simulink model "Simu_ControlLoop_FixPt"  (Simulink 9.2)
settings: Solver=VariableStepAuto  StartTime=0.0  StopTime=25  MaxStep=50e-6  RelTol=1e-3
PreLoadFcn:
  | InitTPV0;
values from neighbouring files (symbols this model uses):
  Imax = 4.4    [InitTPV0.m]
  Kelec = -place(Ae,Be,Pole_elec_desiree)    [InitTPV0.m]
  Kmeca = place(Am,Bm,Pole_meca_desiree)    [InitTPV0.m]
  Ts = 50e-6    (= 5e-05)    [InitTPV0.m]
  Vmax = 24    [InitTPV0.m]
  Wmax = 350    [InitTPV0.m]
undefined symbols (not defined in the file or in its folder): DiscIntNeverNeededParam
libraries: simulink x1
settings Model: Creator=romaindelpoux  LastModifiedBy=rdelpoux
settings SolverCC: ZeroCrossControl=DisableAll  AlgebraicLoopSolver=LineSearch
settings DataIOCC: LimitDataPoints=off  SaveFormat=Dataset  SignalLoggingSaveFormat=Dataset
settings OptimizationCC: LifeSpan=auto
settings DebuggingCC: UnderspecifiedInitializationDetection=Simplified  MergeDetectMultiDrivingBlocksExec=error  FcnCallInpInsideContextMsg=error  StateNameClashWarn=none  SFUnexpectedBacktrackingDiag=error  SFNoUnconditionalDefaultTransitionDiag=error  SFExecutionAtInitializationDiag=warning
settings HardwareCC: ProdBitPerPointer=64  ProdBitPerSizeT=64  ProdBitPerPtrDiffT=64  ProdLargestAtomicFloat=Float  ProdIntDivRoundTo=Zero  ProdEndianess=LittleEndian  ProdWordSize=64  ProdHWDeviceType=Intel->x86-64 (Windows64)
settings ModelReferenceCC: PropagateSignalLabelsOutOfModel=on
settings CodeAppCC: StateflowObjectComments=off
settings GRTTargetCC: TargetLangStandard=C99 (ISO)  GeneratePreprocessorConditionals=Use local settings  CombineOutputUpdateFcns=on  GRTInterface=off
settings ConfigComp: CovMetricSettings=dwe  CovHtmlReporting=off  CovSaveCumulativeToWorkspaceVar=off  CovSaveSingleToWorkspaceVar=off  CovExternalEMLEnable=on

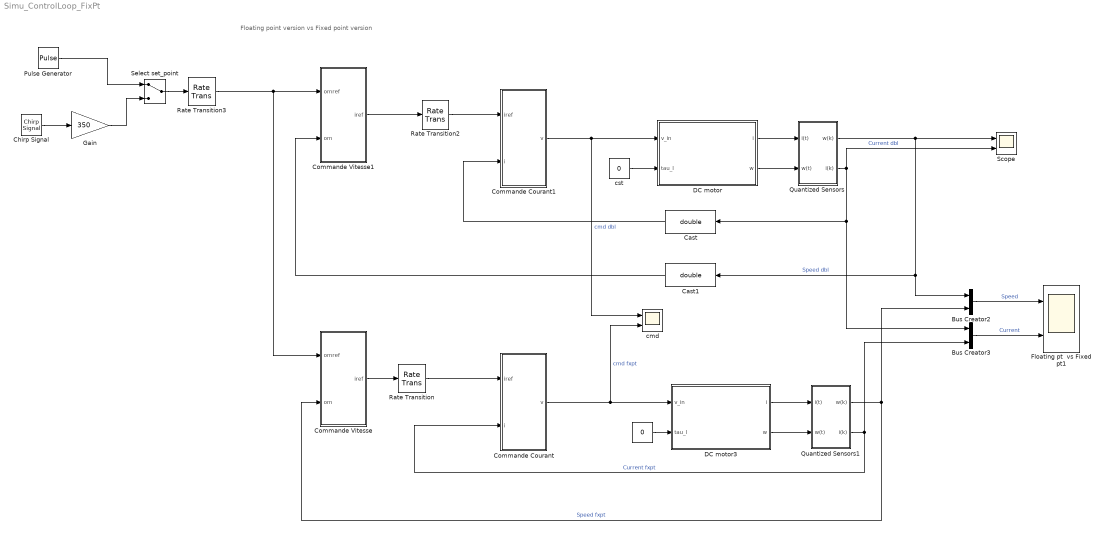
== system Simu_ControlLoop_FixPt ==
  note: Floating point version vs Fixed point version
  " " : Constant  Value=0  OutDataTypeStr=Inherit: Inherit via back propagation
  Bus Creator2 : BusCreator  Inputs=2
  Bus Creator3 : BusCreator  Inputs=2
  Cast : DataTypeConversion  OutDataTypeStr=double
  Cast1 : DataTypeConversion  OutDataTypeStr=double
  Chirp Signal : simulink/Sources/Chirp Signal  f1=0.1  T=20  f2=5
  Commande Courant : Subsystem
  Commande Courant1 : Subsystem
  Commande Vitesse : Subsystem
  Commande Vitesse1 : Subsystem
  DC motor : Subsystem  mask(Motor PRAVALUX MPM4-0002){R=1.22, L=0.0027, Kphi=0.061, J=0.22e-3, F=.0001, C0=-0.032, mod=0.25*0}
      mask prompts: R "Resistance (R) in Ohms"; L "Inductance (L) in H"; Kphi "Back EMF (Kphi) in V/rad/s"; J "J in kgm²"; F "F in N/rad/s"; mod "BEMF modulation (default: 0.25, 0 for off)"
      mask help:
      | Continuous time Model for PRAVALUX MPM4 DC motor
      | Caracteristics: 24V DC, 90W, 5.2A, 3000RPM
      |
      | It is a 2nd order model made of two intertwinned system:
      | one 1st order electrical system and one 1st order mechanical system.
      |
      | Modulation on the BEMF can be added to fit with motor current ripple measured
      |
      | Look under mask (Ctrl-U) to see the model
      mask Display:
      | color('green');
      | image('MotorPravalux.png');
      | %port_label('input',1,'DC');
      | %port_label('output',1,'BEMF');
  DC motor3 : Subsystem  mask(Motor PRAVALUX MPM4-0002){R=1.22, L=0.0027, Kphi=0.061, J=0.22e-3, F=.0001, C0=-0.032, mod=0.25*0}
      mask prompts: R "Resistance (R) in Ohms"; L "Inductance (L) in H"; Kphi "Back EMF (Kphi) in V/rad/s"; J "J in kgm²"; F "F in N/rad/s"; mod "BEMF modulation (default: 0.25, 0 for off)"
      mask help:
      | Continuous time Model for PRAVALUX MPM4 DC motor
      | Caracteristics: 24V DC, 90W, 5.2A, 3000RPM
      |
      | It is a 2nd order model made of two intertwinned system:
      | one 1st order electrical system and one 1st order mechanical system.
      |
      | Modulation on the BEMF can be added to fit with motor current ripple measured
      |
      | Look under mask (Ctrl-U) to see the model
      mask Display:
      | color('green');
      | image('MotorPravalux.png');
      | %port_label('input',1,'DC');
      | %port_label('output',1,'BEMF');
  Floating pt  vs Fixed pt1 : Scope  NumInputPorts=2
  Gain : Gain  Gain=350  OutDataTypeStr=Inherit: Inherit via back propagation
  Pulse Generator : DiscretePulseGenerator  PulseType=Time based  Amplitude=200  PulseWidth=50  PhaseDelay=0.5  SampleTime=-1
  Quantized Sensors : Subsystem
  Quantized Sensors1 : Subsystem
  Rate Transition : RateTransition  Deterministic=off  OutPortSampleTime=50e-6
  Rate Transition2 : RateTransition  Deterministic=off
  Rate Transition3 : RateTransition  Deterministic=off
  Scope : Scope  NumInputPorts=2
  Select set_point : ManualSwitch
  cmd : Scope  NumInputPorts=2
  cst : Constant  Value=0
  wires:
  Commande Vitesse/1(iref) -> Rate Transition/1
  DC motor3/1(i) -> Quantized Sensors1/1(i(t))
  DC motor3/2(w) -> Quantized Sensors1/2(w(t))
  Rate Transition/1 -> Commande Courant/1(iref)
  " "/1 -> DC motor3/2(tau_l)
  Rate Transition2/1 -> Commande Courant1/1(iref)
  Cast/1 -> Commande Courant1/2(i)
  Cast1/1 -> Commande Vitesse1/2(om)
  Rate Transition3/1 -> Commande Vitesse/1(omref), Commande Vitesse1/1(omref)
  DC motor/1(i) -> Quantized Sensors/1(i(t))
  Commande Vitesse1/1(iref) -> Rate Transition2/1
  Pulse Generator/1 -> Select set_point/1
  Select set_point/1 -> Rate Transition3/1
  Gain/1 -> Select set_point/2
  cst/1 -> DC motor/2(tau_l)
  DC motor/2(w) -> Quantized Sensors/2(w(t))
  Chirp Signal/1 -> Gain/1
  Bus Creator3/1 -> Floating pt  vs Fixed pt1/2  "Current"
  Bus Creator2/1 -> Floating pt  vs Fixed pt1/1  "Speed"
  Quantized Sensors/2(i(k)) -> Bus Creator3/1, Cast/1, Scope/2  "Current dbl"
  Quantized Sensors/1(w(k)) -> Bus Creator2/1, Cast1/1, Scope/1  "Speed dbl"
  Quantized Sensors1/2(i(k)) -> Bus Creator3/2, Commande Courant/2(i)  "Current fxpt"
  Quantized Sensors1/1(w(k)) -> Bus Creator2/2, Commande Vitesse/2(om)  "Speed fxpt"
  Commande Courant1/1(v) -> cmd/1, DC motor/1(v_in)  "cmd dbl"
  Commande Courant/1(v) -> cmd/2, DC motor3/1(v_in)  "cmd fxpt"

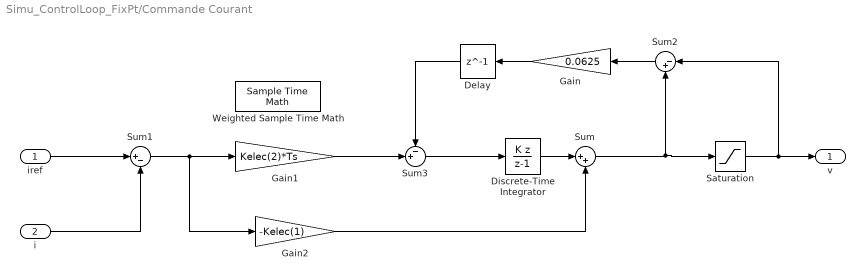
== system Simu_ControlLoop_FixPt/Commande Courant ==
  iref : Inport
  i : Inport  Port=2
  Delay : Delay  DelayLength=1  InitialCondition=0
  Discrete-Time Integrator : DiscreteIntegrator  IntegratorMethod=Accumulation: Backward Euler  SampleTime=.00005  OutMax=Vmax*2  OutDataTypeStr=fixdt(1,32)  SaturateOnIntegerOverflow=on  ICPrevOutput=DiscIntNeverNeededParam  ICPrevScaledInput=DiscIntNeverNeededParam
  Gain : Gain  Gain=0.0625  OutDataTypeStr=Inherit: Inherit via back propagation  SaturateOnIntegerOverflow=on
  Gain1 : Gain  Gain=Kelec(2)*Ts  OutMax=2*Imax*Kelec(2)*Ts  OutDataTypeStr=fixdt(1,16)  SaturateOnIntegerOverflow=on
  Gain2 : Gain  Gain=-Kelec(1)  OutMax=Vmax  OutDataTypeStr=fixdt(1,16)  SaturateOnIntegerOverflow=on
  Saturation : Saturate  UpperLimit=Vmax  LowerLimit=-Vmax
  Sum : Sum  Inputs=|++  OutMax=Vmax*2  OutDataTypeStr=fixdt(1,16)  SaturateOnIntegerOverflow=on
  Sum1 : Sum  Inputs=|+-  OutDataTypeStr=fixdt(1,16,12)  SaturateOnIntegerOverflow=on
  Sum2 : Sum  Inputs=|-+  OutDataTypeStr=Inherit: Same as first input
  Sum3 : Sum  Inputs=-+|  OutDataTypeStr=Inherit: Same as accumulator  SaturateOnIntegerOverflow=on  InputSameDT=on
  Weighted Sample Time Math : SampleTimeMath  TsampMathOp=*  weightValue=Kelec(2)  TsampMathImp=Offline Scaling Adjustment
  v : Outport
  wires:
  iref/1 -> Sum1/1
  i/1 -> Sum1/2
  Sum1/1 -> Gain1/1, Gain2/1
  Gain1/1 -> Sum3/2
  Gain2/1 -> Sum/2
  Sum/1 -> Saturation/1, Sum2/2
  Saturation/1 -> v/1, Sum2/1
  Discrete-Time Integrator/1 -> Sum/1
  Sum3/1 -> Discrete-Time Integrator/1
  Sum2/1 -> Gain/1
  Gain/1 -> Delay/1
  Delay/1 -> Sum3/1

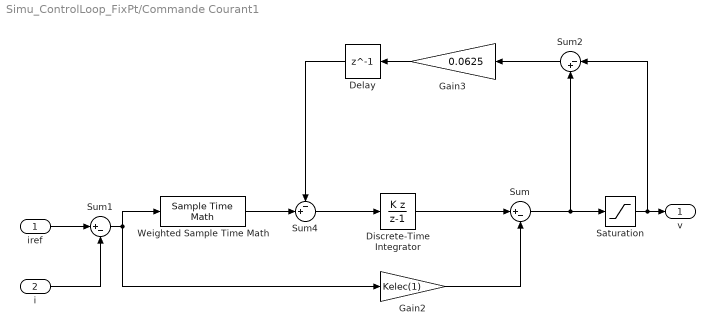
== system Simu_ControlLoop_FixPt/Commande Courant1 ==
  iref : Inport
  i : Inport  Port=2
  Delay : Delay  DelayLength=1  InitialCondition=0
  Discrete-Time Integrator : DiscreteIntegrator  IntegratorMethod=Accumulation: Backward Euler  SampleTime=-1  ICPrevOutput=DiscIntNeverNeededParam  ICPrevScaledInput=DiscIntNeverNeededParam
  Gain2 : Gain  Gain=Kelec(1)
  Gain3 : Gain  Gain=0.0625
  Saturation : Saturate  UpperLimit=Vmax  LowerLimit=-Vmax
  Sum : Sum  Inputs=|+-
  Sum1 : Sum  Inputs=|+-
  Sum2 : Sum  Inputs=|-+  OutDataTypeStr=Inherit: Same as accumulator
  Sum4 : Sum  Inputs=-+|
  Weighted Sample Time Math : SampleTimeMath  TsampMathOp=*  weightValue=Kelec(2)  TsampMathImp=Offline Scaling Adjustment
  v : Outport
  wires:
  Saturation/1 -> v/1, Sum2/1
  Sum/1 -> Saturation/1, Sum2/2
  iref/1 -> Sum1/1
  i/1 -> Sum1/2
  Gain2/1 -> Sum/2
  Sum1/1 -> Gain2/1, Weighted Sample Time Math/1
  Sum4/1 -> Discrete-Time Integrator/1
  Gain3/1 -> Delay/1
  Delay/1 -> Sum4/1
  Discrete-Time Integrator/1 -> Sum/1
  Sum2/1 -> Gain3/1
  Weighted Sample Time Math/1 -> Sum4/2

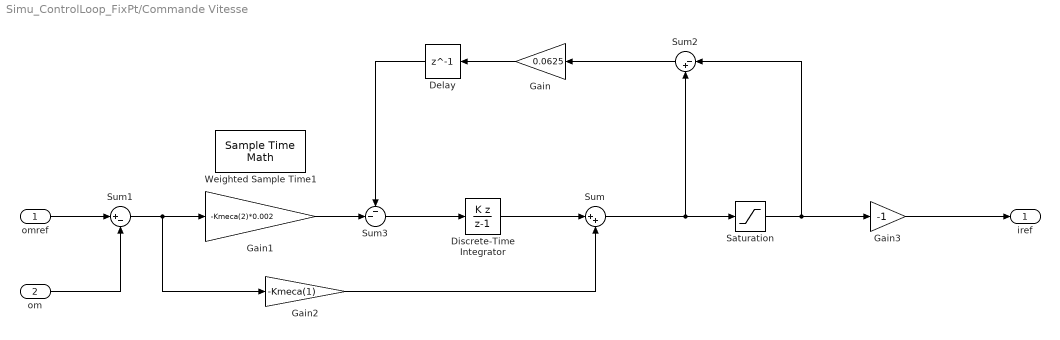
== system Simu_ControlLoop_FixPt/Commande Vitesse ==
  omref : Inport  OutMax=Wmax  OutDataTypeStr=fixdt(1,16)
  om : Inport  Port=2
  Delay : Delay  DelayLength=1  InitialCondition=0
  Discrete-Time Integrator : DiscreteIntegrator  IntegratorMethod=Accumulation: Backward Euler  SampleTime=.002  OutMin=0  OutMax=Imax*2  OutDataTypeStr=fixdt(1,32)  SaturateOnIntegerOverflow=on  ICPrevOutput=DiscIntNeverNeededParam  ICPrevScaledInput=DiscIntNeverNeededParam
  Gain : Gain  Gain=0.0625  OutDataTypeStr=Inherit: Inherit via back propagation  SaturateOnIntegerOverflow=on
  Gain1 : Gain  Gain=-Kmeca(2)*0.002  OutMin=0  OutMax=abs(Wmax * Kmeca(2) * 0.002)  OutDataTypeStr=fixdt(1,16)
  Gain2 : Gain  Gain=-Kmeca(1)  OutMin=-Imax*2  OutMax=Imax*2  OutDataTypeStr=fixdt(1,16)  SaturateOnIntegerOverflow=on
  Gain3 : Gain  Gain=-1  OutMin=-Imax  OutMax=Imax  SaturateOnIntegerOverflow=on  OutDataTypeStr=Inherit: Same as input
  Saturation : Saturate  UpperLimit=Imax  LowerLimit=-Imax
  Sum : Sum  Inputs=|++  OutMin=-Imax  OutMax=Imax*2  OutDataTypeStr=fixdt(1,16)  SaturateOnIntegerOverflow=on
  Sum1 : Sum  Inputs=|+-  OutMin=-Wmax*2  OutMax=Wmax*2  OutDataTypeStr=fixdt(1,16)
  Sum2 : Sum  Inputs=|-+  OutDataTypeStr=Inherit: Same as accumulator
  Sum3 : Sum  Inputs=--|  OutDataTypeStr=Inherit: Same as accumulator  SaturateOnIntegerOverflow=on  InputSameDT=on
  Weighted Sample Time1 : SampleTimeMath  TsampMathOp=*  weightValue=-Kmeca(2)  TsampMathImp=Offline Scaling Adjustment
  iref : Outport
  wires:
  omref/1 -> Sum1/1
  Gain2/1 -> Sum/2
  om/1 -> Sum1/2
  Sum/1 -> Sum2/2, Saturation/1
  Saturation/1 -> Sum2/1, Gain3/1
  Sum3/1 -> Discrete-Time Integrator/1
  Sum2/1 -> Gain/1
  Gain3/1 -> iref/1
  Sum1/1 -> Gain1/1, Gain2/1
  Gain/1 -> Delay/1
  Delay/1 -> Sum3/1
  Discrete-Time Integrator/1 -> Sum/1
  Gain1/1 -> Sum3/2

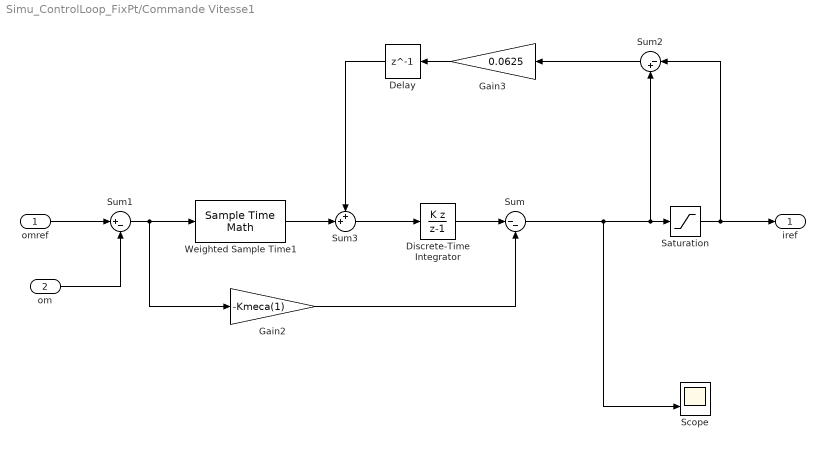
== system Simu_ControlLoop_FixPt/Commande Vitesse1 ==
  omref : Inport
  om : Inport  Port=2
  Delay : Delay  DelayLength=1  InitialCondition=0
  Discrete-Time Integrator : DiscreteIntegrator  IntegratorMethod=Accumulation: Backward Euler  SampleTime=-1  ICPrevOutput=DiscIntNeverNeededParam  ICPrevScaledInput=DiscIntNeverNeededParam
  Gain2 : Gain  Gain=-Kmeca(1)
  Gain3 : Gain  Gain=0.0625  OutDataTypeStr=Inherit: Inherit via back propagation
  Saturation : Saturate  UpperLimit=Imax  LowerLimit=-Imax
  Scope : Scope  NumInputPorts=2
  Sum : Sum  Inputs=|--
  Sum1 : Sum  Inputs=|+-
  Sum2 : Sum  Inputs=|-+  OutDataTypeStr=Inherit: Same as accumulator
  Sum3 : Sum  Inputs=++|
  Weighted Sample Time1 : SampleTimeMath  TsampMathOp=*  weightValue=Kmeca(2)
  iref : Outport
  wires:
  Delay/1 -> Sum3/1
  Gain3/1 -> Delay/1
  Weighted Sample Time1/1 -> Sum3/2
  Sum3/1 -> Discrete-Time Integrator/1
  Discrete-Time Integrator/1 -> Sum/1
  Saturation/1 -> iref/1, Sum2/1
  Sum/1 -> Scope/2, Sum2/2, Saturation/1
  om/1 -> Sum1/2
  omref/1 -> Sum1/1
  Sum1/1 -> Gain2/1, Weighted Sample Time1/1
  Sum2/1 -> Gain3/1
  Gain2/1 -> Sum/2

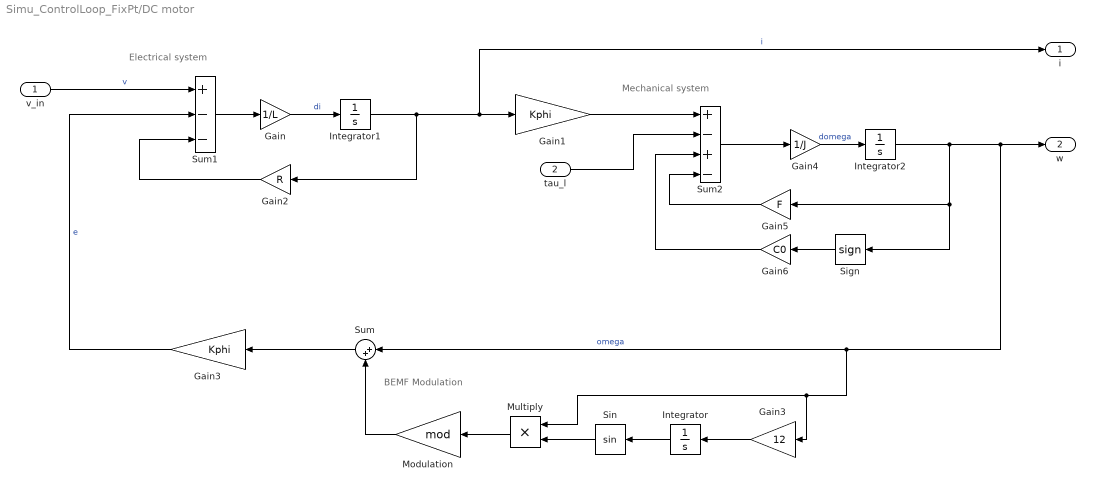
== system Simu_ControlLoop_FixPt/DC motor ==
  note: Electrical system
  note: Mechanical system
  note: BEMF Modulation
  v_in : Inport  SampleTime=0
  tau_l : Inport  Port=2
  Gain : Gain  Gain=1/L
  Gain1 : Gain  Gain=Kphi
  Gain2 : Gain  Gain=R
  Gain3 : Gain  Gain=12
  "Gain3  " : Gain  Gain=Kphi
  Gain4 : Gain  Gain=1/J
  Gain5 : Gain  Gain=F
  Gain6 : Gain  Gain=C0
  Integrator : Integrator  WrapState=on
  Integrator1 : Integrator
  Integrator2 : Integrator
  Modulation : Gain  Gain=mod
  Multiply : Product
  Sign : Signum
  Sin : Trigonometry
  Sum : Sum  Inputs=|++
  Sum1 : Sum  Inputs=+--
  Sum2 : Sum  Inputs=+-+-
  i : Outport
  w : Outport  Port=2
  wires:
  Gain1/1 -> Sum2/1
  Gain4/1 -> Integrator2/1  "domega"
  Sum2/1 -> Gain4/1
  Gain5/1 -> Sum2/4
  Integrator2/1 -> Gain5/1, Sign/1, Multiply/1, Gain3/1, Sum/1, w/1  "omega"
  Sign/1 -> Gain6/1
  Gain6/1 -> Sum2/3
  tau_l/1 -> Sum2/2
  "Gain3  "/1 -> Sum1/2  "e"
  Gain2/1 -> Sum1/3
  v_in/1 -> Sum1/1  "v"
  Integrator1/1 -> Gain1/1, i/1, Gain2/1  "i"
  Gain/1 -> Integrator1/1  "di"
  Sum1/1 -> Gain/1
  Gain3/1 -> Integrator/1
  Integrator/1 -> Sin/1
  Multiply/1 -> Modulation/1
  Modulation/1 -> Sum/2
  Sum/1 -> "Gain3  "/1
  Sin/1 -> Multiply/2

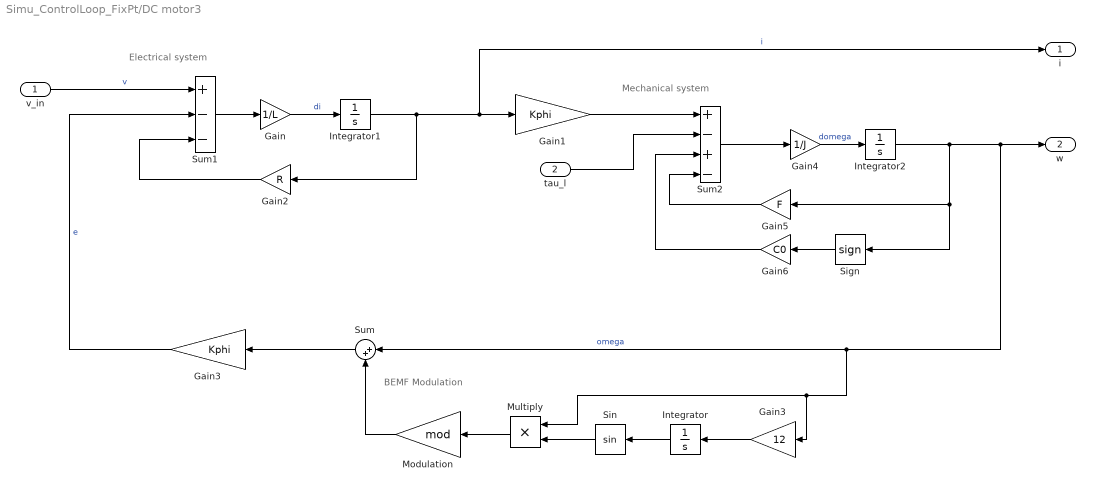
== system Simu_ControlLoop_FixPt/DC motor3 ==
  note: Electrical system
  note: Mechanical system
  note: BEMF Modulation
  v_in : Inport  SampleTime=0
  tau_l : Inport  Port=2
  Gain : Gain  Gain=1/L
  Gain1 : Gain  Gain=Kphi
  Gain2 : Gain  Gain=R
  Gain3 : Gain  Gain=12
  "Gain3  " : Gain  Gain=Kphi
  Gain4 : Gain  Gain=1/J
  Gain5 : Gain  Gain=F
  Gain6 : Gain  Gain=C0
  Integrator : Integrator  WrapState=on
  Integrator1 : Integrator
  Integrator2 : Integrator
  Modulation : Gain  Gain=mod
  Multiply : Product
  Sign : Signum
  Sin : Trigonometry
  Sum : Sum  Inputs=|++
  Sum1 : Sum  Inputs=+--
  Sum2 : Sum  Inputs=+-+-
  i : Outport
  w : Outport  Port=2
  wires:
  Gain1/1 -> Sum2/1
  Gain4/1 -> Integrator2/1  "domega"
  Sum2/1 -> Gain4/1
  Gain5/1 -> Sum2/4
  Integrator2/1 -> Gain5/1, Sign/1, Multiply/1, Gain3/1, Sum/1, w/1  "omega"
  Sign/1 -> Gain6/1
  Gain6/1 -> Sum2/3
  tau_l/1 -> Sum2/2
  "Gain3  "/1 -> Sum1/2  "e"
  Gain2/1 -> Sum1/3
  v_in/1 -> Sum1/1  "v"
  Integrator1/1 -> Gain1/1, i/1, Gain2/1  "i"
  Gain/1 -> Integrator1/1  "di"
  Sum1/1 -> Gain/1
  Gain3/1 -> Integrator/1
  Integrator/1 -> Sin/1
  Multiply/1 -> Modulation/1
  Modulation/1 -> Sum/2
  Sum/1 -> "Gain3  "/1
  Sin/1 -> Multiply/2

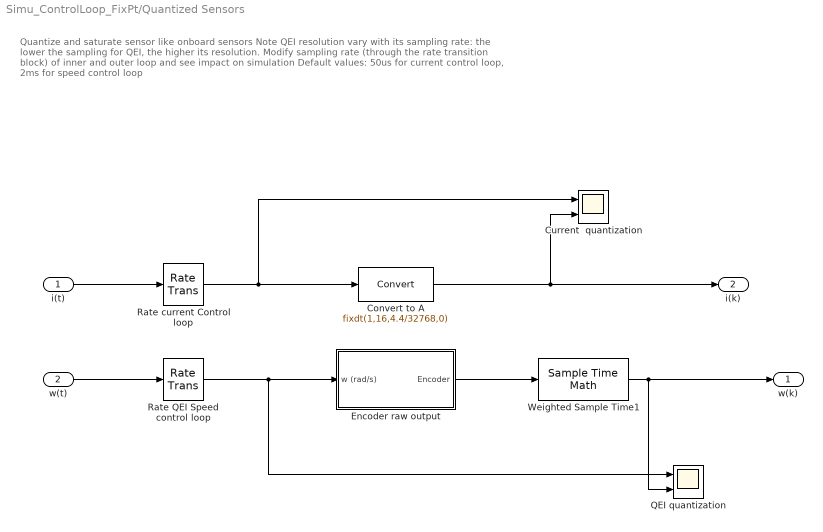
== system Simu_ControlLoop_FixPt/Quantized Sensors ==
  note: Quantize and saturate sensor like onboard sensors
      |
      | Note QEI resolution vary with its sampling rate:
      | the lower the sampling for QEI, the higher its resolution.
      |
      | Modify sampling rate (through the rate transition block) of inner and outer loop and see impact on simulation
      |
      | Default values: 50us for current control loop, 2ms for speed control loop
  i(t) : Inport
  w(t) : Inport  Port=2
  Convert to A : DataTypeConversion  OutDataTypeStr=fixdt(1,16,4.4/32768,0)  SaturateOnIntegerOverflow=on  LockScale=on
  Current  quantization : Scope  NumInputPorts=2
  Encoder raw output : Subsystem
  QEI quantization : Scope  NumInputPorts=2
  Rate QEI Speed control loop : RateTransition  Deterministic=off  OutPortSampleTime=.002
  Rate current Control loop : RateTransition  Deterministic=off  OutPortSampleTime=50e-6
  Weighted Sample Time1 : SampleTimeMath  TsampMathOp=/  weightValue=1000/pi  TsampMathImp=Offline Scaling Adjustment
  w(k) : Outport
  i(k) : Outport  Port=2
  wires:
  Weighted Sample Time1/1 -> w(k)/1, QEI quantization/2
  Rate current Control loop/1 -> Current  quantization/1, Convert to A/1
  i(t)/1 -> Rate current Control loop/1
  w(t)/1 -> Rate QEI Speed control loop/1
  Convert to A/1 -> Current  quantization/2, i(k)/1
  Rate QEI Speed control loop/1 -> Encoder raw output/1(w (rad/s)), QEI quantization/1
  Encoder raw output/1(Encoder) -> Weighted Sample Time1/1

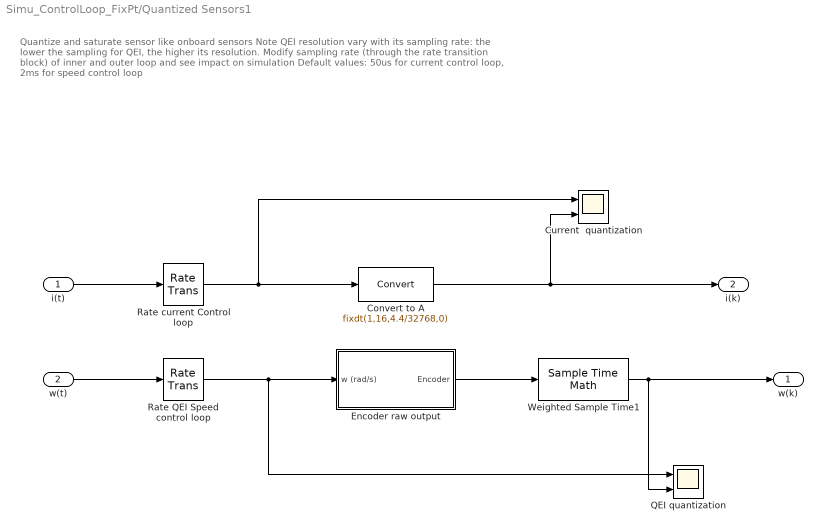
== system Simu_ControlLoop_FixPt/Quantized Sensors1 ==
  note: Quantize and saturate sensor like onboard sensors
      |
      | Note QEI resolution vary with its sampling rate:
      | the lower the sampling for QEI, the higher its resolution.
      |
      | Modify sampling rate (through the rate transition block) of inner and outer loop and see impact on simulation
      |
      | Default values: 50us for current control loop, 2ms for speed control loop
  i(t) : Inport
  w(t) : Inport  Port=2
  Convert to A : DataTypeConversion  OutDataTypeStr=fixdt(1,16,4.4/32768,0)  SaturateOnIntegerOverflow=on  LockScale=on
  Current  quantization : Scope  NumInputPorts=2
  Encoder raw output : Subsystem
  QEI quantization : Scope  NumInputPorts=2
  Rate QEI Speed control loop : RateTransition  Deterministic=off  OutPortSampleTime=.002
  Rate current Control loop : RateTransition  Deterministic=off  OutPortSampleTime=50e-6
  Weighted Sample Time1 : SampleTimeMath  TsampMathOp=/  weightValue=1000/pi  TsampMathImp=Offline Scaling Adjustment
  w(k) : Outport
  i(k) : Outport  Port=2
  wires:
  Encoder raw output/1(Encoder) -> Weighted Sample Time1/1
  Rate QEI Speed control loop/1 -> QEI quantization/1, Encoder raw output/1(w (rad/s))
  Convert to A/1 -> i(k)/1, Current  quantization/2
  w(t)/1 -> Rate QEI Speed control loop/1
  i(t)/1 -> Rate current Control loop/1
  Rate current Control loop/1 -> Convert to A/1, Current  quantization/1
  Weighted Sample Time1/1 -> QEI quantization/2, w(k)/1

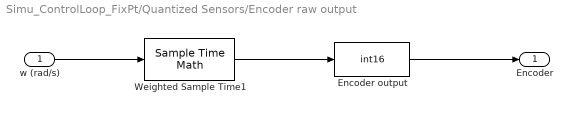
== system Simu_ControlLoop_FixPt/Quantized Sensors/Encoder raw output ==
  w (rad/s) : Inport
  Encoder output : DataTypeConversion  OutDataTypeStr=int16  SaturateOnIntegerOverflow=on  LockScale=on
  Weighted Sample Time1 : SampleTimeMath  TsampMathOp=*  weightValue=1000/pi
  Encoder : Outport
  wires:
  Weighted Sample Time1/1 -> Encoder output/1
  Encoder output/1 -> Encoder/1
  w (rad/s)/1 -> Weighted Sample Time1/1

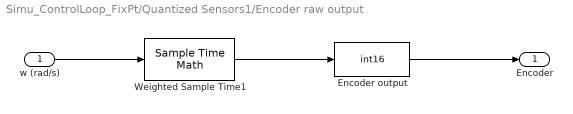
== system Simu_ControlLoop_FixPt/Quantized Sensors1/Encoder raw output ==
  w (rad/s) : Inport
  Encoder output : DataTypeConversion  OutDataTypeStr=int16  SaturateOnIntegerOverflow=on  LockScale=on
  Weighted Sample Time1 : SampleTimeMath  TsampMathOp=*  weightValue=1000/pi
  Encoder : Outport
  wires:
  w (rad/s)/1 -> Weighted Sample Time1/1
  Encoder output/1 -> Encoder/1
  Weighted Sample Time1/1 -> Encoder output/1
